simulink model "SAC_simulink"  (R2025b)
settings: Solver=ode4  StartTime=0.0  StopTime=180  FixedStep=0.01  RelTol=1e-3
values from neighbouring files (symbols this model uses):
  action_limits_lower = 0.88    [main_SAC.m]
  action_limits_upper = 1.07    [main_SAC.m]
  b0 = (1-t)^3    [ph7_teta_vincolato_new.m]
  k = Num_k./(Den_k + 1e-6)    [ph7_teta_vincolato_new.m]
  par_phys = struct    [main_SAC.m]    (also in test_all_agents_random_training_domain.m)
  rigeneration_step_s = 300    [main_SAC.m]
  T = resultsTable(ok, :)    [test_all_agents_random_training_domain.m]
  target = [0; 0; 0]    [test_all_agents_random_training_domain.m]
  Ts = 150    [main_SAC.m]    (also in test_all_agents_random_training_domain.m)
undefined symbols (not defined in the file or in its folder): delay, delta_a_max, h_max, h_min, k0_target, k1_target, k_L, max_idx, mean_vertical_velocity, meters_end_zf, r_max, r_min, s_f_time, t1_max_rad, t1_min_rad, t_step, wc, X0, yaw_max, yaw_min
libraries: slctrl_adaptive x3, aerolibobsolete x1, aerolibasang x1, simulink x1, aerolibatmos2 x1, rllib x1
(part 2 of 2)

== matlab function SAC_simulink/SIGNAL_PROCESSING /Reward_Assembly_SubSys/MATLAB Function ==
  data: heading_error input; reward output; DeltaDistanceToTarget input; z_f_error input; flush_flag input; isFirstStep input; IsDone_virtual input; R_acc output; frozen output; R_acc input; frozen input
function [reward, R_acc, frozen] = fun_reward_assembly( ...
    heading_error, DeltaDistanceToTarget, z_f_error, ...
    flush_flag, isFirstStep, IsDone_virtual, R_acc, frozen)
    
    BASELINE_REWARD = 0;
    
    % 1. Salviamo il valore appena entrato
    R_acc_in = R_acc; 
    
    % 2. Inizializzazione 
    if isFirstStep || (R_acc_in == BASELINE_REWARD)
        R_acc  = BASELINE_REWARD; 
        frozen = 0; % 0 = Casse aperte, si accumula
    end
    
    % 3. Logica di Accumulo
    if frozen == 0 % Se la reward finale NON è ancora stata aggiunta
        
        if IsDone_virtual == 0
            % VOLO NORMALE
            R_acc = R_acc + DeltaDistanceToTarget + heading_error;
            
        else
            % EPISODIO FINITO
            if z_f_error ~= 0
                R_acc = R_acc + z_f_error;
                frozen = 1; % 1 = Casse chiuse! La transazione è avvenuta.
            end
        end
    end
    
    % 4. BLOCCO FLUSH 
    if flush_flag && ~isFirstStep && (R_acc_in ~= BASELINE_REWARD)
        reward = R_acc;
        R_acc  = 0;
        
        % Manteniamo la cassaforte chiusa se l'episodio è finito
        if IsDone_virtual || frozen == 1
            frozen = 1;
        else
            frozen = 0;
        end
    else
        reward = R_acc;
    end
end


% function [reward, R_acc, frozen] = fun_reward_assembly( ...
%     heading_error, DeltaDistanceToTarget, z_f_error, ...
%     flush_flag, isFirstStep, IsDone_virtual, R_acc, frozen)
% 
%     BASELINE_REWARD = -15000;
% 
%     % 1. Salviamo il valore appena entrato dal blocco Memory
%     R_acc_in = R_acc; 
% 
%     % 2. Inizializzazione Blindata (La tua versione!)
%     % Scatta se Simulink ci dice che è il primo step 
%     % OPPURE se il blocco Memory inietta fisicamente la baseline (-2000)
%     if isFirstStep || (R_acc_in == BASELINE_REWARD)
%         R_acc  = BASELINE_REWARD; 
%         frozen = 0;
%     end
% 
%     % 3. Macchina a Stati per l'Accumulo (Per non perdere z_f_error)
%     if frozen == 0
%         % STATO 0: Volo normale
%         R_acc = R_acc + DeltaDistanceToTarget + heading_error;
% 
%         if IsDone_virtual
%             if z_f_error ~= 0
%                 R_acc = R_acc + z_f_error;
%                 frozen = 2; 
%             else
%                 frozen = 1; % Aspetta z_f_error al prossimo step
%             end
%         end
% 
%     elseif frozen == 1
%         % STATO 1: In attesa della penalità finale
%         if z_f_error ~= 0
%             R_acc = R_acc + z_f_error;
%             frozen = 2; 
%         end
% 
%     elseif frozen == 2
%         % STATO 2: Sigillato, non accumulare più nulla
%     end
% 
%     % 4. BLOCCO FLUSH (La tua versione blindata!)
%     % Svuota l'accumulatore SOLO se c'è il flag e non siamo a -2000
%     if flush_flag && ~isFirstStep && (R_acc_in ~= BASELINE_REWARD)
%         reward = R_acc;
%         R_acc  = 0;
% 
%         % Manteniamo il congelamento se l'episodio è finito
%         if IsDone_virtual || frozen == 2
%             frozen = 2;
%         else
%             frozen = 0;
%         end
%     else
%         reward = R_acc;
%     end
% end

== matlab function SAC_simulink/GNC & Environment/GNC/MATLAB Function9 ==
  settings: updateMethod=DISCRETE  sampleTime=0.01
  data: flag_act output; sim_time input; act output; interval input
function [flag_act, act] = activator(sim_time, interval)

    persistent next_trigger_time % flag

    if isempty(next_trigger_time)
        next_trigger_time = 0;
    end
    
    act = -1;
    flag_act = 0;

    if sim_time >= next_trigger_time
        act = 1;
        flag_act = 1;
        next_trigger_time = next_trigger_time + interval;
    end

end

== matlab function SAC_simulink/SIGNAL_PROCESSING /Reward_Assembly_SubSys/error_signals/Subsystem/MATLAB Function1 ==
  data: pos input; DeltaDistanceToTarget output; target input; isFirstStep input; r_prev input; r_prev output
function [DeltaDistanceToTarget, r_prev]= fun_compute_DDTT(pos, target, isFirstStep, r_prev)
    if isempty(r_prev) || isFirstStep
        r_prev = sqrt((pos(1)-target(1))^2 + (pos(2)-target(2))^2);
        DeltaDistanceToTarget = 0;
        return
    end
    r_now = sqrt((pos(1)-target(1))^2 + (pos(2)-target(2))^2);
    DeltaDistanceToTarget = (r_prev - r_now);
    r_prev = r_now;
end

== matlab function SAC_simulink/SIGNAL_PROCESSING /Reward_Assembly_SubSys/error_signals/Subsystem1/MATLAB Function1 ==
  data: err_psi input; heading_error output
function heading_error = sum_heading_error_fun(err_psi)
    % Convertiamo l'errore in gradi (valore assoluto)
    err_deg = abs(err_psi) * 180 / pi; 
    
    % --- PARAMETRI ---
    A = 20;      % Penalità massima desiderata
    T = 110.0;     % Soglia di attivazione in gradi
    P = 8;        % Potenza (determina quanto è piatto l'inizio e brusco il crollo)
    
    % --- FUNZIONE MATEMATICA CONTINUA ---
    heading_error = -A * tanh( (err_deg / T)^P );
end


% function heading_error  = sum_heading_error_fun (err_psi)
% 
%     heading_error = -3*tanh(1.3 * err_psi/pi)^2;
% 
% end

== matlab function SAC_simulink/SIGNAL_PROCESSING /Reward_Assembly_SubSys/error_signals/Error z_f -> correct landing indicator/MATLAB Function ==
  data: target input; pos input; r output
function r = radius_pos2target(target, pos)
r = sqrt((pos(1)-target(1))^2 + (pos(2)-target(2))^2);
end

== matlab function SAC_simulink/SIGNAL_PROCESSING /Reward_Assembly_SubSys/error_signals/Error z_f -> correct landing indicator/MATLAB Function5 ==
  data: r input; pos input; z_f output; flag input; flag_turned input; flag_z_f output; flag_z_f_in input; z_f_in input
function [z_f, flag_z_f] = fun_z_f(r, pos, flag, flag_turned, flag_z_f_in, z_f_in)
    % Se è già lockato, restituisci il valore che avevi in ingresso (memoria).
    % Questo manterrà anche l'eventuale penalità intatta per tutto il resto dell'episodio.
    if flag_z_f_in == 1
        z_f = z_f_in;   % Mantieni il valore precedente
        flag_z_f = 1;   % Mantieni il lock
        return;
    end
    
    % Valori di default se nessuna condizione è soddisfatta
    z_f = 0;
    flag_z_f = 0;
    
    % --- CONTROLLO CONDIZIONI E PENALITA' ---
    calcola_reward = false;
    penalizza = false;
    
    % Valutiamo le condizioni in modo indipendente per evitare che un flag 
    % positivo nasconda un malus contemporaneo.
    condizione_base  = (flag == 1 || flag == 2);
    condizione_malus = (flag_turned == 1 || flag == 3);
    
    % Se si verifica una qualsiasi condizione di attivazione nel raggio d'azione
    if (condizione_base || condizione_malus) && (r <= 15)
        calcola_reward = true;
        
        % La penalità ha priorità assoluta
        if condizione_malus
            penalizza = true;
        end
    end
    
    % --- CALCOLO DELLA FUNZIONE z_f ---
    if calcola_reward
        z = -1 * pos(3);
        
        % --- PARAMETRI NUOVA REWARD SMOOTH ---
        % Banda utile
        z_low  = 7;
        z_high = 15;
        z_ref  = 10;

        % Limiti globali richiesti
        z_min = -600;
        z_max =  600;

        % Livelli reward
        R_edge     = 302;    % reward esatta a z = -600 e z = +600
        R_shoulder = 5000;   % reward appena fuori banda
        R_plateau  = 11000;  % reward interna quasi piatta
        R_peak     = 1000;   % bonus centrale -> massimo totale 12000

        % Parametri di forma
        alpha = 4;          % ripidità della finestra morbida
        delta = 2;        % quanto la transizione "sborda" fuori dalla banda
        sigma = 10;         % larghezza del picco centrale
        kL    = 300;         % decadimento lato sinistro
        kR    = 300;         % decadimento lato destro

        sig = @(x) 1 ./ (1 + exp(-x));

        % Finestra morbida: ~1 dentro [7,15], ~0 fuori, senza gradino
        w = sig(alpha * (z - (z_low  - delta))) - sig(alpha * (z - (z_high + delta)));
        w = min(max(w, 0), 1);

        % Shaping esterno normalizzato:
        % s = 1 al bordo della banda, s = 0 a z = z_min o z = z_max
        if z < z_low
            d    = z_low - z;
            dmax = z_low - z_min;
            s    = (exp(-d / kL) - exp(-dmax / kL)) / (1 - exp(-dmax / kL));
        elseif z > z_high
            d    = z - z_high;
            dmax = z_max - z_high;
            s    = (exp(-d / kR) - exp(-dmax / kR)) / (1 - exp(-dmax / kR));
        else
            s = 1;
        end

        s = min(max(s, 0), 1);

        % Reward esterna
        r_out = R_edge + (R_shoulder - R_edge) * s;

        % Reward interna con piccolo picco attorno a z_ref
        center = exp(-((z - z_ref) / sigma)^2);
        r_in   = R_plateau + R_peak * center;

        % Blending liscio tra esterno e interno
        z_f_temp = r_out + w .* (r_in - r_out);

        % Cap massimo richiesto
        z_f_temp = min(z_f_temp, 12000);
        
        % --- APPLICAZIONE PENALITÀ ---
        % Se i flag attivi richiedono una penalità, dimezziamo il risultato calcolato
        if penalizza
            z_f_temp = z_f_temp * 0.5;
        end
        
        % Assegna il valore finale e attiva il lock per i prossimi step
        z_f = z_f_temp;
        flag_z_f = 1; 
    end
end


% function [z_f, flag_z_f] = fun_z_f_fixed(r, pos, flag, flag_turned, flag_z_f_in, z_f_in)
%     % Se è già lockato, restituisci il valore che avevi in ingresso (memoria)
%     if flag_z_f_in == 1
%         z_f = z_f_in;   % Mantieni il valore precedente
%         flag_z_f = 1;   % Mantieni il lock
%         return;
%     end
% 
%     % Valori di default se nessuna condizione è soddisfatta
%     z_f = 0;
%     flag_z_f = 0;
% 
%     % Controllo condizioni di attivazione lock immediato
%     if flag_turned == 1 || flag == 3
%         z_f = 0; % Oppure un valore specifico richiesto per queste flag
%         flag_z_f = 1;
%         return;
%     end
% 
%     % Calcolo della funzione z_f
%     if (flag == 1 || flag == 2) && r <= 15
%         z = -1 * pos(3);
% 
%         % --- PARAMETRI MODIFICABILI ---
%         Peak   = 12000;  % Valore massimo della forza
%         z_peak = 10;     % Quota in cui si ha il picco
%         L_up   = 15.3;   % Pendenza della discesa verso l'alto
%         L_down = 22.6;   % Pendenza della discesa verso il basso
% 
%         z_up   = 20;     % Punto in cui inizia il tratto lineare superiore
%         z_down = -5;     % Punto in cui inizia il tratto lineare inferiore
% 
%         z_max  = 100;    % Quota dove la forza si azzera in alto
%         z_min  = -75;    % Quota dove la forza si azzera in basso
%         % ------------------------------
% 
%         if z >= z_max
%             z_f = 0;
% 
%         elseif z >= z_up
%             % Raccordo lineare superiore (dinamico)
%             V_up = Peak * (1 - tanh((z_up - z_peak) / L_up));
%             z_f = V_up * (z_max - z) / (z_max - z_up);
% 
%         elseif z >= z_peak
%             % Curva morbida superiore (tanh)
%             z_f = Peak * (1 - tanh((z - z_peak) / L_up));
% 
%         elseif z > z_down
%             % Curva morbida inferiore (tanh)
%             z_f = Peak * (1 - tanh((z_peak - z) / L_down));
% 
%         elseif z >= z_min
%             % Raccordo lineare inferiore (dinamico)
%             V_down = Peak * (1 - tanh((z_peak - z_down) / L_down));
%             z_f = V_down * (z - z_min) / (z_down - z_min);
% 
%         else
%             z_f = 0;
%         end
% 
%         z_f = max(0, z_f);
%         flag_z_f = 1; % Qui il lock viene attivato per il prossimo step
%     end
% end





% function z_f = fun_z_f_error(pos, flag, target, flag_turned)
% 
%     % 1. Dichiara le variabili come memoria interna al blocco
%     persistent internal_state_turned;
%     persistent locked_z_f; 
%     persistent has_locked; 
% 
%     % 2. Inizializzazione (scatta solo al primissimo avvio di Simulink)
%     if isempty(internal_state_turned)
%         internal_state_turned = 0;
%         locked_z_f = 0; 
%         has_locked = 0; 
%     end
% 
%     % ========================================================
%     % 2.5 AUTO-RESET PER NUOVO EPISODIO (IL FIX DEL BUG)
%     % Se siamo in volo (flag = 0) ma la funzione è "bloccata", 
%     % significa che è finito un episodio vecchio e ne sta iniziando
%     % uno nuovo. Resettiamo le memorie!
%     if flag == 0 && has_locked == 1
%         internal_state_turned = 0;
%         locked_z_f = 0;
%         has_locked = 0;
%     end
%     % ========================================================
% 
%     % 3. LATCH LOGICO
%     if flag_turned == 1
%         internal_state_turned = 1;
%     end
% 
%     % 4. SHORT-CIRCUIT
%     if has_locked == 1
%         z_f = locked_z_f;
%         return;
%     end
% 
%     % 5. Calcolo della distanza orizzontale (raggio)
%     r = sqrt((pos(1)-target(1))^2 + (pos(2)-target(2))^2);
% 
%     % 6. Macchina a stati
%     if flag == 0
%         current_z_f = 0;
% 
%     elseif internal_state_turned == 1 
%         current_z_f = 0;
% 
%     elseif flag == 1 || flag == 2  % ATTERRATO / IN ZONA
% 
%         if r < 15
%             % Estraiamo l'altezza z
%             z_height = pos(3); 
%             max_reward = 12000;
% 
%             % Parametri di pendenza aggiornati
%             scale_fast = 1.2;  % Molto veloce sotto i 10m
%             scale_slow = 5.0;  % Più lenta sopra i 10m
% 
%             if z_height >= 10
%                 % ZONA SUPERIORE: z >= 10 (discesa lenta)
%                 current_z_f = max_reward * (1 - tanh((z_height - 10) / scale_slow));
% 
%             else
%                 % ZONA INFERIORE: z < 10 (discesa molto veloce)
%                 current_z_f = max_reward * (1 - tanh((10 - z_height) / scale_fast));
%             end
% 
%             % Tronchiamo a zero per evitare valori negativi
%             if current_z_f < 0
%                 current_z_f = 0;
%             end
% 
%         else
%             current_z_f = 0;
%         end
% 
%     elseif flag == 3 % FALLIMENTO / TEMPO SCADUTO
%         current_z_f = 1000;
% 
%     else
%         current_z_f = 0;
%     end
% 
%     % 7. CONGELAMENTO DELLA REWARD
%     % Al primo step in cui il flag diventa 1, congela il valore calcolato sopra.
%     if flag ~= 0 || internal_state_turned == 1
%         locked_z_f = current_z_f;
%         has_locked = 1;
%     end
% 
%     % 8. Assegnazione dell'output
%     % Questo fa uscire correttamente la reward appena calcolata nel singolo istante.
%     z_f = current_z_f;
% 
% end

% function reward = reward_fun(pos, flag)
%     if flag == 1
%         Z = pos(3);
%         % penalità quadratica su Z, niente termine r
%         reward = -(Z^2);
%     elseif flag == 2
%         % episodio scartato (timeout) → penalità fissa grande
%         reward = -1000;
%        elseif flag == 3
%         % episodio scartato (timeout) → penalità fissa grande
%         reward = -10000; 
%     else
%         reward = 0;
%     end
% end

== matlab function SAC_simulink/SIGNAL_PROCESSING /Observation vector costruction/h_normalizzation/MATLAB Function ==
  data: h input; h_n output; h_min input; h_max input
function h_n = fcn(h, h_min, h_max)
h_n = (h - h_min) / (h_max - h_min);

== matlab function SAC_simulink/SIGNAL_PROCESSING /Observation vector costruction/Subsystem1/MATLAB Function ==
  data: yaw input; yaw_n output; yaw_min input; yaw_max input
function yaw_n = fun_yaw_n(yaw, yaw_min, yaw_max)
    % 1. Saturazione (Clipping)
    % Se il valore supera i limiti, viene bloccato a yaw_max o yaw_min
    yaw_clipped = max(min(yaw, yaw_max), yaw_min);
    
    % 2. Normalizzazione
    % Dividiamo per il valore assoluto del massimo
    % per ottenere un range tra -1 e +1
    yaw_n = yaw_clipped / abs(yaw_max);
end

== matlab function SAC_simulink/SIGNAL_PROCESSING /Observation vector costruction/Subsystem/MATLAB Function1 ==
  data: pos input; r_n output; target input; r_min input; r_max input; h_min input; h_max input; h_n output
function [r_n, h_n] = fun_pos_norm(pos, target, r_min, r_max, h_min, h_max)
    % 1. Calcolo distanza euclidea sul piano X-Y (Raggio)
    r = sqrt((pos(1)-target(1))^2 + (pos(2)-target(2))^2);
    
    % 2. Estrazione altezza (Z) dalla terza componente di pos
    h = pos(3);
    
    % 3. Saturazione (Clipping) per evitare valori fuori dai range [0, 1]
    r_clipped = max(min(r, r_max), r_min);
    h_clipped = max(min(h, h_max), h_min);
    
    % 4. Normalizzazione Min-Max (Output tra 0 e 1)
    r_n = (r_clipped - r_min) / (r_max - r_min);
    h_n = (h_clipped - h_min) / (h_max - h_min);
end

== matlab function SAC_simulink/SIGNAL_PROCESSING /Observation vector costruction/Subsystem4/MATLAB Function ==
  data: err_psi input; err_psi_norm output
function err_psi_norm = fun_error_psi_normalizzed(err_psi)

err_psi_norm = err_psi / pi;

== matlab function SAC_simulink/GNC & Environment/Environment/Subsystem/MATLAB Function1 ==
  data: alpha input; Ma output; delta_a input; b input; omb input; rho input; S input; Va input; clphi input; clp input; cldelta_a input; cndelta_a input; cm0 input; cm_alpha input; cm_q input; cn_r input; c input; euler input
function Ma = aeroMoment(alpha,delta_a,b,omb,rho,S,Va,clphi,clp,cldelta_a,cndelta_a,cm0,cm_alpha,cm_q,cn_r,c,euler)
% this function computes the aerodynamic moment of the parafoil

% INPUT
% alpha         : attack angle                                     [rad]
% delta_a       : asymmetric deflection                            [m]
% b             : wingspan                                         [m]
% omb           : body angular velocity                       [3x1][rad/s]
% rho           : air density                                      [kg/m^3]
% S             : aerodynamic surface                              [m^2] 
% Va            : airspeed vector                                  [m/s]
% clphi         : cl roll derivative                               [-]
% clp           : cl roll rate derivative                          [-] 
% cldelta_a     : roll coefficient derivative                      [-]
% cndelta_a     : yaw coefficient derivative                       [-]
% cm0           : zero alpha aero moment coefficient               [-]
% cm_alpha      : derivative of the moment coefficient             [-]
% cm_q          : moment coefficient derivative pitch rate         [-] 
% cn_r          : yaw coefficient derivative wrt to roll rate      [-] 
% c             : aerodynamic choord                               [m]
% euler         : roll,pitch,yaw                              [3x1][rad]


% roll angle extraction
phi = euler(1);
% angular velocity extraction 
p = omb(1);
q = omb(2);
r = omb(3);
% asymetric deflection normalization 
delta_a_bar = delta_a/0.05;
% aerodynamic moment computation 
Ma = 0.5*rho*S*(Va^2)*[clphi*b*phi + clp*(b^2)*p/(2*Va) + cldelta_a*delta_a_bar*b;
        cm0*c + cm_alpha*alpha*c + cm_q*(c^2)*q/(2*Va) ;
        cn_r*(b^2)*r/(2*Va) + cndelta_a*b*delta_a_bar];

end

== matlab function SAC_simulink/SIGNAL_PROCESSING /Reward_Assembly_SubSys/Reward_FlushFlag_Generator/MATLAB Function1 ==
  data: t input; flush_flag output; Ts input; t_step input
function flush_flag = fun_flush_flag(t, Ts, t_step)
    % Ts sample time agente  [s]
    % t_step sample time controllore [s]
    
    % mod(t, Ts) < tolleranza → siamo su un multiplo di 25s
    % t > 0 → esclude t=0 (primo step, R_acc è già 0 per isFirstStep)
    flush_flag = double( (mod(t, Ts) < t_step * 0.5) && (t > 0) );
end

== matlab function SAC_simulink/SIGNAL_PROCESSING /Trigger_IsDone_real/MATLAB Function ==
  data: t input; IsDone_real output; Ts input; t_step input; IsDone_virtual input; t_trigger input; armed input; t_trigger output; armed output
function [IsDone_real, t_trigger, armed] = fun_delay_isdone(t, Ts, t_step, IsDone_virtual, t_trigger, armed)
    
    % Se IsDone_virtual scatta per la prima volta, armiamo il timer e non lo disarmiamo più
    if IsDone_virtual && ~armed
        % Calcola il prossimo step dell'agente. 
        next_agent_step = ceil((t + t_step*0.1) / Ts) * Ts;
        
        % Imposta il momento esatto in cui far scattare la fine (+ 2 secondi di margine)
        t_trigger = next_agent_step - 0.1;
        
        % armed passa a 1 e ci rimarrà per sempre
        armed = 1;
    end
    
    % IsDone_real diventa 1 quando t raggiunge t_trigger.
    % Siccome 't' continua a crescere e 'armed' non viene più azzerato, 
    % IsDone_real rimarrà ancorato a 1 per tutto il resto della simulazione.
    IsDone_real = double( armed && (t >= t_trigger) );

end

== matlab function SAC_simulink/GNC & Environment/GNC/MATLAB Function13 ==
  data: prev_idx input; prev_idx_clean output; old_idx input; act input
function prev_idx_clean = fcn(prev_idx, old_idx, act)
    if prev_idx < 200
        prev_idx_clean = prev_idx;
    else
        prev_idx_clean = 200;
    end

    if act == 1
        prev_idx_clean = 1;
    end

end

== matlab function SAC_simulink/GNC & Environment/GNC/MATLAB Function18 ==
  data: V input; act input; X_start input; path_xy output; t_start input; target input; t1_min_rad input; t1_max_rad input; L_actual output; comp_time output; t1_opt_deg output; cp_real_out output; w_coeffs_out output; geom_info output; k0_target input; k1_target input; k_L input
function [path_xy, L_actual, comp_time, t1_opt_deg, cp_real_out, w_coeffs_out, geom_info] = fcn(V, act, X_start, t_start, target, t1_min_rad, t1_max_rad, k0_target, k1_target, k_L)
%#codegen

% Dichiariamo la funzione esterna (quella che hai modificato per restituire scalari)
coder.extrinsic('ph7_teta_vincolato_new');

%% 1. DEFINIZIONE MEMORIA (PERSISTENT)
persistent p_path_xy p_L_actual p_comp_time p_t1_opt_deg p_cp_real_out p_w_coeffs_out p_geom_info

if isempty(p_path_xy)
    p_path_xy = zeros(200, 2); % ONLY for debugging
    p_L_actual = 0;
    p_comp_time = 0;
    p_t1_opt_deg = 0;
    p_cp_real_out = zeros(8, 2);
    p_w_coeffs_out = zeros(4, 2);
    p_geom_info = zeros(1, 2);
end

%% 2. LOGICA DI TRIGGER
if act == 1
    % A. Logica Fisica
    if abs(V(3)) < 1e-6
        V_free_fall = 5;
    else
        V_free_fall = abs(V(3));
    end
    dt_flight = abs(X_start(3)) / V_free_fall; 
    V_horiz = sqrt(V(1)^2 + V(2)^2);
    
    if V_horiz < 1e-3
        L_target = 10;
        theta0_ph = 0;
    else
        L_base = dt_flight * V_horiz;
        L_target = L_base * k_L;
        theta0_ph = atan2(t_start(2), t_start(1)); 
    end
    P0_ph = [X_start(1), X_start(2)];       
    P1_ph = [target(1), target(2)]; 
    
    % B. Pre-inizializzazione variabili output (Fondamentale per Simulink)
    % Simulink deve sapere tipi e dimensioni prima della chiamata extrinsic
    curve_pts_cx = complex(zeros(1, 200)); 
    cp_real_cx = complex(zeros(1, 8));
    w_coeffs_cx = complex(zeros(1, 4));
    angle_chord = 0;
    dist_chord = 0;
    L_val = 0;
    Time_val = 0;
    t1_val = 0;
    
    % C. Chiamata DIRETTA alla funzione modificata
    % Nota: L_val, Time_val, t1_val corrispondono agli ultimi 3 output scalari
    [curve_pts_cx, cp_real_cx, w_coeffs_cx, angle_chord, dist_chord, L_val, Time_val, t1_val] = ...
        ph7_teta_vincolato_new(...
        P0_ph, P1_ph, theta0_ph, t1_min_rad, t1_max_rad, ...
        k0_target,k1_target, L_target, ...
        'verbose', false, 'diagnostics', false, 'use_exact', true);
    
    % D. Aggiornamento Memoria
    p_path_xy(:,1) = real(curve_pts_cx).'; 
    p_path_xy(:,2) = imag(curve_pts_cx).'; 
    
    p_cp_real_out(:,1) = real(cp_real_cx).';
    p_cp_real_out(:,2) = imag(cp_real_cx).';
    
    p_w_coeffs_out(:,1) = real(w_coeffs_cx).';
    p_w_coeffs_out(:,2) = imag(w_coeffs_cx).';
    
    p_geom_info = [angle_chord, dist_chord];
    
    p_L_actual = L_val;
    p_comp_time = Time_val;
    p_t1_opt_deg = t1_val * (180/pi);
end

%% 3. ASSEGNAZIONE OUTPUT
path_xy      = p_path_xy; % NOT ACTIVELY USED -> ONLY FOR DEBUGGING
L_actual     = p_L_actual;
comp_time    = p_comp_time;
t1_opt_deg   = p_t1_opt_deg;
cp_real_out  = p_cp_real_out;
w_coeffs_out = p_w_coeffs_out;
geom_info    = p_geom_info;
end

== matlab function SAC_simulink/GNC & Environment/GNC/MATLAB Function19 ==
  data: err_psi output; pos_3d input size=[3 1]; psi_attuale input; path_2d input; L input; psi_des output; idx_target output; prev_idx input
function [err_psi, psi_des, idx_target] = guidance_ground_track(pos_3d, psi_attuale, path_2d, L, prev_idx)
%#codegen
% GUIDANCE_GROUND_TRACK
% Nota: %#codegen è obbligatorio per dire a MATLAB di controllare i tipi statici.
    err_psi = 0;
    psi_des = 0;
    %% 1. Inizializzazione Sicura
    % Definiamo idx_target come scalare double fin da subito.
    idx_target = double(prev_idx); 

    %% 2. Data Slicing
    L_LOOKAHEAD = L;
    pos_2d = pos_3d(1:2); 
    pos_2d = pos_2d(:);
    
    [n_points, cols] = size(path_2d);
    % In simulazione real-time, l'error() ferma tutto. Meglio un dummy check.
    if cols ~= 2
        % Gestione emergenza silenziosa o return safe
        return; 
    end
    
    %% 3. Calcolo Distanze
    diff_vec = path_2d - pos_2d(:)'; 
    dist_sq = sum(diff_vec.^2, 2); 
    L_sq = L_LOOKAHEAD^2;
    
    is_outside = dist_sq > L_sq;
    for i = 1:prev_idx
        is_outside(i) = 0;
    end
    
    % FIX CRITICO 1: Convertiamo in double prima di diff per evitare logici ambigui
    transitions = diff(double(is_outside)); 
    
    % FIX CRITICO 2: Isoliamo l'output di 'find' in una variabile temporanea
    idx_trans_raw = find(transitions == 1, 1, 'first');
    
    %% 4. Logica di Selezione Target
    if ~isempty(idx_trans_raw)
        % FIX CRITICO 3: Accesso esplicito all'elemento (1).
        % Questo rompe il legame "variable-size" e forza uno scalare.
        idx_found = idx_trans_raw(1);
        
        idx_target = double(idx_found);
        
    else
        % FALLBACK LOGIC (La tua logica originale)
        idx_target = double(n_points);
    end
    
    %% 5. Safety Check Finale (Anti-Crash)
    % Se per qualche motivo matematico usciamo dai bounds, clippiamo.
    if idx_target > n_points
        idx_target = double(n_points);
    elseif idx_target < 1
        idx_target = 1.0;
    end
    %idx_target = max(idx_target, double(prev_idx));

    p_target = path_2d(floor(idx_target), :)';
    
    %% 6. Calcolo Heading
    los = p_target - pos_2d;
    psi_des = atan2(los(2), los(1));
    
    %% 7. Output Error
    err_psi = atan2(sin(psi_des - psi_attuale), cos(psi_des - psi_attuale));
end

== matlab function SAC_simulink/GNC & Environment/GNC/MATLAB Function20 ==
  data: v input; L output; T input
function L = lookahead_distance(v, T)   
    v_or = sqrt(v(1)^2+v(2)^2);
    L = v_or*T;
end

== matlab function SAC_simulink/GNC & Environment/GNC/MATLAB Function21 ==
  data: X0 input; idx input; X_start output; path_xy input; V0 input; t_start output; T input
function [X_start, t_start] = aiming_point(X0, idx, path_xy, V0, T)
    
    % Inizializza il vettore colonna 3x1 per il punto di mira
    X_start = zeros(3,1);
    
    % 1. VETTORE DIREZIONE (t_start):
    % Punta dalla tua posizione orizzontale (X,Y) verso il waypoint (X,Y)
    t_start = [path_xy(idx,:)]' - [X0(1); X0(2)];
    
    % 2. MIRA ORIZZONTALE:
    % Copia le coordinate X e Y del waypoint
    X_start(1:2,1) = path_xy(idx,:);
    
    % 3. MIRA VERTICALE PREDITTIVA:
    % Calcola la quota stimata dopo T secondi
    X_start(3,1) = X0(3) + V0(3)*T;

end

== matlab function SAC_simulink/GNC & Environment/Environment/Subsystem/MATLAB Function ==
  data: S input; rho input; vb input; Fa output; Va input; alpha input; delta_a input; cl0 input; cl_alpha input; cd0 input; cd_alpha_2 input; cd_delta_a input; cL_delta_a input; E output
function [Fa,E]  = aeroForce(S,rho,vb,Va,alpha,delta_a,cl0,cl_alpha,cd0,cd_alpha_2,cd_delta_a,cL_delta_a)
% this function computes the aerodynamic forces [d,q,l] in body frame

% INPUTS
% S            : aerodynamic surface        [m^2]
% rho          : air density                [kg/m^3]
% vb           : body velocity vector [3x1] [m/s]
% Va           : airspeed vector      [3x1] [m/s]
% alpha        : attack angle               [rad]
% delta_a      : asymetric deflection       [m]
% cl0          : zero alpha lift coeff      [-]
% cl_alpha     : lift coefficient derivative[-]
% cd0          : zero alpha drag coeff      [-]
% cd_alpha_2   : quadratic drag coefficient [-]
% cd_delta_a   : drag coeff asymm deflection[-]
% cL_delta_a   : lift coeff asymm deflection[-]
% 
% OUTPUT 
% Fa           : aerodynamic force     [3x1] [N]


% body velocity extraction 
u = vb(1);
v = vb(2);
w = vb(3);

% normalization of the asymetric deflection
delta_a_bar = abs(delta_a/0.05);

% computation of the aerodynamic force
Fa = 0.5*rho*S*Va*(cl0 + cl_alpha*alpha + cL_delta_a*delta_a_bar)*[w;0;-u]... 
        - 0.5*rho*S*Va*(cd0 + cd_alpha_2*(alpha^2) + cd_delta_a*delta_a_bar)*[u;v;w];
% questo non ha senso non guardarlo
E = abs(Fa(3)/Fa(1));

end

== matlab function SAC_simulink/GNC & Environment/Environment/MATLAB Function ==
  data: vb input; Va output; dcm input; W input; Va_n output
function [Va,Va_n] = velocity(vb,dcm,W)
% -------------------------------------------------------------------------
% vb   = Velocità del velivolo in coordinate BODY (3x1) [m/s]
% dcm  = Direzione Coseni Matrix (3x3), trasforma vettori da Earth a BODY
% W    = Vettore velocità del vento in coordinate Earth (3x1) [m/s]
%
% Va   = Norm(a) del vettore di velocità relativa all’aria (airspeed) [m/s]
% Va_n = Vettore di airspeed in coordinate BODY (3x1) [m/s]
% -------------------------------------------------------------------------

% Calcolo del vettore di airspeed (BODY) sottraendo il vento in BODY
Va_n = vb - dcm * W;
% Va_n = vb - W;

% Calcolo del modulo (airspeed scalare)
Va = norm(Va_n);

end

== matlab function SAC_simulink/GNC & Environment/Environment/MATLAB Function1 ==
  data: dcm input; fg output; m input
function fg = gravity(dcm,m)



fg = (m*9.81*dcm*[0;0;1]);

== matlab function SAC_simulink/SIGNAL_PROCESSING /Observation vector costruction/Subsystem2/MATLAB Function2 ==
  data: pos input; r_n output; target input; r_min input; r_max input
function r_n = fun_r_n(pos, target, r_min, r_max)
r = sqrt((pos(1)-target(1))^2 + (pos(2)-target(2))^2);
    r_n    = (r     - r_min)     / (r_max     - r_min); % normalizzato tra 0 1
end

== matlab function SAC_simulink/GNC & Environment/Environment/MATLAB Function3 ==
  data: u input; y output
function y = fcn(u)

y = sqrt(u(1).^2+u(2).^2);
